simulink model "Problem4"  (R2020a)
settings: Solver=ode15s  StartTime=0.0  StopTime=0.2  RelTol=1e-3
model workspace (MAT data in the model file):
  J = 3.2284e-06
  K = 0.0274
  L = 2.75e-06
  R = 4
  b = 3.5077e-06
settings Model: DataDictionary=motor_data.sldd  Creator=aishw  LastModifiedBy=aishw
settings DebuggingCC: AlgebraicLoopMsg=none

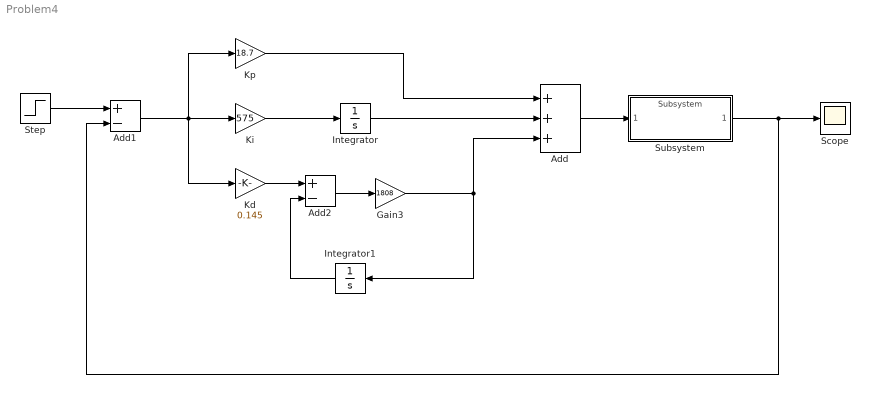
== system Problem4 ==
  Add : Sum  Inputs=+++
  Add1 : Sum  Inputs=+-
  Add2 : Sum  Inputs=+-
  Gain3 : Gain  Gain=1808
  Integrator : Integrator
  Integrator1 : Integrator
  Kd : Gain  Gain=0.145
  Ki : Gain  Gain=575
  Kp : Gain  Gain=18.7
  Scope : Scope
  Step : Step  Time=0  SampleTime=0
  Subsystem : ModelReference  ModelNameDialog=Subsystem  ModelReferenceVersion=1.2
  wires:
  Subsystem/1 -> Add1/2, Scope/1
  Add2/1 -> Gain3/1
  Ki/1 -> Integrator/1
  Kd/1 -> Add2/1
  Kp/1 -> Add/1
  Integrator/1 -> Add/2
  Integrator1/1 -> Add2/2
  Add1/1 -> Kd/1, Ki/1, Kp/1
  Gain3/1 -> Integrator1/1, Add/3
  Step/1 -> Add1/1
  Add/1 -> Subsystem/1
